simulink model "TST_rx_byte_aligner_32bit"  (R2024a)
settings: Solver=FixedStepDiscrete  StartTime=0.0  StopTime=16  FixedStep=1  RelTol=1e-3
settings Model: Creator=User  LastModifiedBy=Vetaly
settings SolverCC: AlgebraicLoopSolver=TrustRegion
settings DataIOCC: LimitDataPoints=on  SaveFormat=Array  SignalLoggingSaveFormat=ModelDataLogs  SaveOutput=off  SaveTime=off  ReturnWorkspaceOutputs=off
settings OptimizationCC: BlockReduction=off  ConditionallyExecuteInputs=off  DefaultParameterBehavior=Inlined  ExpressionDepthLimit=2147483647  LifeSpan=inf
settings DebuggingCC: AlgebraicLoopMsg=error  ArtificialAlgebraicLoopMsg=none  UnderspecifiedInitializationDetection=Classic  MergeDetectMultiDrivingBlocksExec=none  InheritedTsInSrcMsg=none  SingleTaskRateTransMsg=error  IntegerOverflowMsg=none  FcnCallInpInsideContextMsg=warning  ModelReferenceSymbolNameMessage=none  StateNameClashWarn=warning  SFUnexpectedBacktrackingDiag=warning  SFNoUnconditionalDefaultTransitionDiag=warning  SFExecutionAtInitializationDiag=none  IntegerSaturationMsg=none  ArithmeticOperatorsInVariantConditions=warning
settings HardwareCC: ProdBitPerPointer=32  ProdBitPerSizeT=32  ProdBitPerPtrDiffT=32  ProdLargestAtomicFloat=None  ProdIntDivRoundTo=Undefined  ProdEndianess=Unspecified  ProdWordSize=32  ProdHWDeviceType=ASIC/FPGA->ASIC/FPGA  ProdEqTarget=off
settings ModelReferenceCC: EnableRefExpFcnMdlSchedulingChecks=on  ModelReferenceMinAlgLoopOccurrences=on  PropagateSignalLabelsOutOfModel=off
settings SFSimCC: SimUseLocalCustomCode=off  SimParseCustomCode=off  CustomCodeUndefinedFunction=UseInterfaceOnly
settings RTWCC: RTWVerbose=off  RTWUseLocalCustomCode=off  RTWCompilerOptimization=on  GPUComputeCapability=3.5  DLArmComputeVersion=19.05
settings CodeAppCC: StateflowObjectComments=on
settings GRTTargetCC: TargetLangStandard=C89/C90 (ANSI)  CombineOutputUpdateFcns=off  GRTInterface=on
settings ConfigComp: CovMetricSettings=dw  CovSaveCumulativeToWorkspaceVar=on  CovSaveSingleToWorkspaceVar=on  CovExternalEMLEnable=off

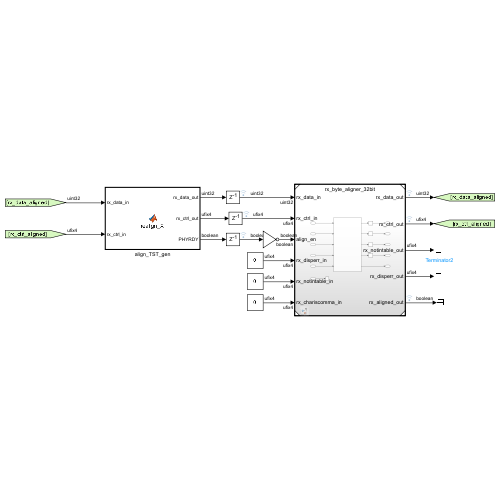
[thumbnail: Simulink's stored preview of the top-level diagram]
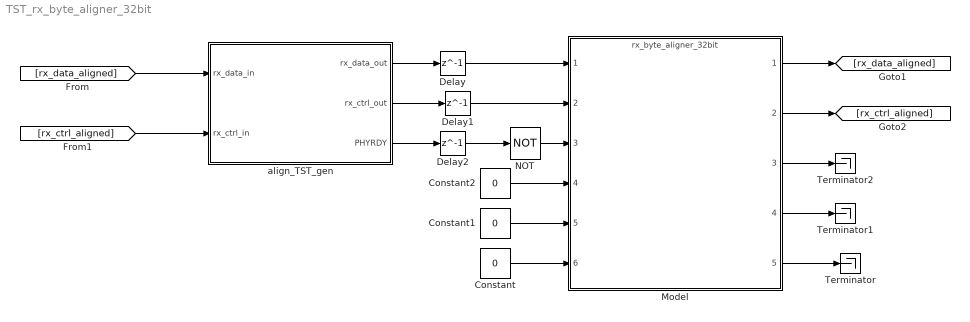
== system TST_rx_byte_aligner_32bit ==
  Constant : Constant  Value=0  OutDataTypeStr=fixdt(0,4,0)  SampleTime=-1
  Constant1 : Constant  Value=0  OutDataTypeStr=fixdt(0,4,0)  SampleTime=-1
  Constant2 : Constant  Value=0  OutDataTypeStr=fixdt(0,4,0)  SampleTime=-1
  Delay : Delay  DelayLength=1
  Delay1 : Delay  DelayLength=1
  Delay2 : Delay  DelayLength=1
  Model : ModelReference  ModelNameDialog=rx_byte_aligner_32bit.slx  SimulationMode=Normal  ModelReferenceVersion=10.102
  NOT : Logic  Operator=NOT  IconShape=distinctive  AllPortsSameDT=off  OutDataTypeStr=boolean
  Terminator : Terminator
  Terminator1 : Terminator
  Terminator2 : Terminator
  align_TST_gen : MATLAB Function  TreatAsAtomicUnit=on
  wires:
  align_TST_gen/1(rx_data_out) -> Delay/1
  align_TST_gen/2(rx_ctrl_out) -> Delay1/1
  align_TST_gen/3(PHYRDY) -> Delay2/1
  Model/1 -> [rx_data_aligned]
  [rx_data_aligned] -> align_TST_gen/1(rx_data_in)
  Model/2 -> [rx_ctrl_aligned]
  [rx_ctrl_aligned] -> align_TST_gen/2(rx_ctrl_in)
  Delay/1 -> Model/1
  Delay1/1 -> Model/2
  Delay2/1 -> NOT/1
  Model/5 -> Terminator/1
  NOT/1 -> Model/3
  Constant2/1 -> Model/4
  Constant1/1 -> Model/5
  Constant/1 -> Model/6
  Model/4 -> Terminator1/1
  Model/3 -> Terminator2/1

== matlab function TST_rx_byte_aligner_32bit/align_TST_gen ==
  settings: sampleTime=1
  settings: fimath=|
      | fimath(...
      | 'RoundMode', 'floor',...
      | 'OverflowMode', 'wrap',...
      | 'ProductMode', 'FullPrecision', 'ProductWordLength', 16,...
      | 'SumMode', 'FullPrecision', 'SumWordLength', 16,...
      | 'CastBeforeSum', true)
  data: rx_data_in input; rx_data_out output; rx_ctrl_out output; rx_ctrl_in input; PHYRDY output
function [rx_data_out, rx_ctrl_out, PHYRDY] = realign_X(rx_data_in, rx_ctrl_in)
fm = fimath('OverflowMode','Wrap');

COMMA_BYTE = 0xBC;
% COMMA_BYTE = '0xBC';

persistent states counter PHYRDY_r
if isempty(states)
    states = fi(0,0,2,0,fm);
    counter = fi(0,0,2,0,fm);
    % PHYRDY_r = false;
end

PHYRDY = false;

switch states
    case 0
        rx_data_out = uint32(0x4ABC7B4A);
        rx_ctrl_out = fi(4,0,4,0,fm);

        % if (counter<2)
        if (rx_data_in==0x7B4A4ABC && rx_ctrl_in==1)
            if (counter<2)
            % states(1) = 0;
                counter = fi(counter + 1, 0, counter.WordLength, 0, fm);
            else
                states(1) = 1;
                counter = fi(0, 0, counter.WordLength, 0, fm);
                PHYRDY_r = true;
                PHYRDY = true;
            end
        else
            counter = fi(0, 0, counter.WordLength, 0, fm);
            states(1) = 0;
        end
        % counter = fi(counter + 1, 0, counter.WordLength, 0, fm);

    case 1
        rx_ctrl_out = fi(0,0,4,0,fm);
        PHYRDY = true;
        switch counter
            case 0
                rx_data_out = uint32(0x11007B4A);
            case 1
                rx_data_out = uint32(0x55443322);
            case 2
                rx_data_out = uint32(0x99887766);
            otherwise
                rx_data_out = uint32(0xDDCCBBAA);
        end
        if (counter<3)
            states(1) = 1;
        else
            states(1) = 2;
        end
        counter = fi(counter + 1, 0, counter.WordLength, 0, fm);
    otherwise
        PHYRDY = true;
        % rx_data_out = uint32(0);
        % rx_ctrl_out = fi(0,0,4,0,fm);

        rx_data_out = uint32(0x4A4ABC7B);
        rx_ctrl_out = fi(2,0,4,0,fm);

end
